simulink model "Main_Sim"  (R2020b)
settings: Solver=FixedStepAuto  StartTime=0.0  StopTime=57060  FixedStep=simParams.sample_time_s  RelTol=1e-3  EnableMultiTasking=on
values from neighbouring files (symbols this model uses):
  test_data = struct    [sim_init.m]
undefined symbols (not defined in the file or in its folder): eclipse, elev_gs_rad, elev_targ_rad, FSW_Lib, gnc_mode, gyro_body_radps, gyro_meas_valid, mag_body_T, mag_meas_valid, mekf_3sigma_rad, mekf_bias_radps, mtq_cmd_Am2, photodiodes_A, rwa_cmd_rpm, sc_above_gs, sc_above_targ, sc_body_rates_radps, sc_quat, Sensors_Lib, sgp4_flag, simParams, solar_panel_power_W, sun_meas_ss_deg, sun_meas_valid, target_gen_flag
libraries: dspstat3 x4, gyroscope_lib x3, magnetometer_lib x3, simulink_extras x2, actuators_lib x1, CDH_command_lib x1, Environment_lib x1, MEKF_Conversion_lib x1, MEKF_lib x1, actuator_processing_lib x1, control_command_generation_lib x1, evironmentEstimation_lib x1
settings Model: Creator=devantormey  LastModifiedBy=Zach Daniel
settings DataIOCC: ReturnWorkspaceOutputs=off
settings OptimizationCC: DefaultParameterBehavior=Inlined  UseDivisionForNetSlopeComputation=on  UseFloatMulNetSlope=on  InlineInvariantSignals=on  PassReuseOutputArgsAs=Individual arguments  ZeroExternalMemoryAtStartup=off  ZeroInternalMemoryAtStartup=off  NoFixptDivByZeroProtection=on  EfficientFloat2IntCast=on  LifeSpan=1  OptimizeBlockOrder=speed  DifferentSizesBufferReuse=on  EfficientTunableParamExpr=on
settings DebuggingCC: ParameterTunabilityLossMsg=error  BusObjectLabelMismatch=error  SFUnexpectedBacktrackingDiag=warning  SFNoUnconditionalDefaultTransitionDiag=warning  ArithmeticOperatorsInVariantConditions=warning
settings HardwareCC: ProdBitPerPointer=32  ProdBitPerSizeT=32  ProdBitPerPtrDiffT=32  ProdLargestAtomicInteger=Long  ProdLargestAtomicFloat=Double  ProdWordSize=32  ProdLongLongMode=on  ProdHWDeviceType=NXP->Cortex-M4
settings SFSimCC: SimUseLocalCustomCode=off  MATLABDynamicMemAlloc=off  CustomCodeUndefinedFunction=UseInterfaceOnly
settings RTWCC: Description=Embedded Coder  SystemTargetFile=ert.tlc  TemplateMakefile=ert_default_tmf  GenerateReport=on  RTWUseLocalCustomCode=off  IncludeHyperlinkInReport=on  LaunchReport=on  GenerateTraceInfo=on  GenerateTraceReport=on  GenerateTraceReportSl=on  GenerateTraceReportSf=on  GenerateTraceReportEml=on  GenerateCodeMetricsReport=on
settings CodeAppCC: ForceParamTrailComments=on  IgnoreCustomStorageClasses=off  OperatorAnnotations=on  SimulinkDataObjDesc=on  SFDataObjDesc=on  CustomSymbolStrGlobalVar=rt$N$M  CustomSymbolStrType=$N$M  CustomSymbolStrFcn=$N$M$F  CustomSymbolStrMacro=$N$M  InsertBlockDesc=on
settings ERTTargetCC: GenerateSampleERTMain=on  IncludeMdlTerminateFcn=off  CombineSignalStateStructs=on  SupportComplex=off  SupportContinuousTime=on  SupportNonInlinedSFcns=on  InlinedParameterPlacement=NonHierarchical  ERTCustomFileTemplate=example_file_process.tlc
settings ConfigComp: CovMetricSettings=dw  CovSaveCumulativeToWorkspaceVar=on  CovSaveSingleToWorkspaceVar=on  CovExternalEMLEnable=off

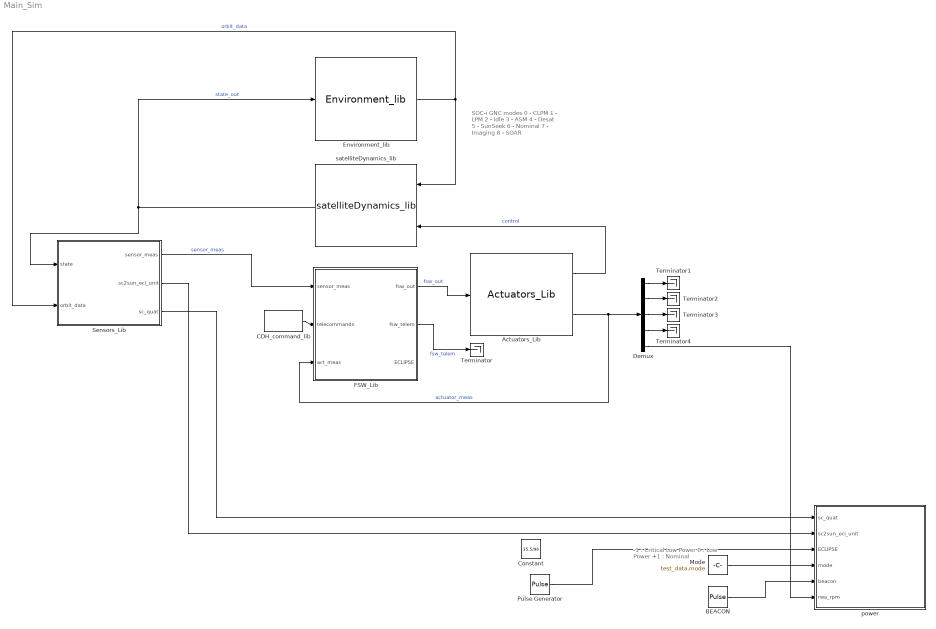
== system Main_Sim ==
  note: SOC-i GNC modes
      | 0 - CLPM
      | 1 - LPM
      | 2 - Idle
      | 3 - ASM
      | 4 - Desat
      | 5 - SunSeek
      | 6 - Nominal
      | 7 - Imaging
      | 8 - SOAR
  note: -1	: Critical Low Power
      |   0	: Low Power
      | +1	: Nominal
  Actuators_Lib : actuators_lib/Actuators_Lib  SystemSampleTime=-1  VariantActivationTime=update diagram  Latency=0  AutoFrameSizeCalculation=off
  BEACON : DiscretePulseGenerator  PulseType=Time based  Period=60  PulseWidth=100 * (1.0 / 60)
  CDH_command_lib : CDH_command_lib/CDH_command_lib  target_lat_deg=target_lat_deg  target_lon_deg=target_lon_deg  target_alt_m=target_alt_m  override_autonomy=0  enable_pointing=off  force_clpm=off  force_lpm=off  enable_img=off  enable_soar=off  triad_override=off  mask{target_lat_deg=44.0, target_lon_deg=-76.5, target_alt_m=0.0, override_autonomy=0, enable_pointing=off, force_clpm=off, force_lpm=off, enable_img=off, enable_soar=off, triad_override=off}
      mask prompts: target_lat_deg "Target Latitude [deg]"; target_lon_deg "Target Longitude [deg]"; target_alt_m "Target Alt [m]"; override_autonomy "Override Autonomous Mode Selection"; enable_pointing "Enable Autonomous Pointing"; force_clpm "CLPM Operating Mode"; force_lpm "LPM Operating Mode"; enable_img "Enable IMG"; enable_soar "Enable SOAR"; triad_override "TRIAD Override"
      mask TypeOptions target_lat_deg: target_lat_deg
      mask TypeOptions target_lon_deg: target_lon_deg
      mask TypeOptions target_alt_m: target_alt_m
      mask TypeOptions override_autonomy: override_autonomy
      mask TypeOptions enable_pointing: enable_pointing
      mask TypeOptions force_clpm: force_clpm
      mask TypeOptions force_lpm: force_lpm
      mask TypeOptions enable_img: enable_img
      mask TypeOptions enable_soar: enable_soar
      mask TypeOptions triad_override: triad_override
      mask DialogControl DescGroupVar Prompt: SOC-i Telecommand Module
      mask DialogControl DescTextVar Prompt: Adjust the parameters that can enter the GNC flight software from the rest of the satellite, including the other subsystems onboard and those that come from the ground station.
  Constant : Constant  Value=35.5/96  VectorParams1D=off
  Demux : Demux  Outputs=[5 4 1 1 4]
  Environment_lib : Environment_lib/Environment_lib  SystemSampleTime=-1  VariantActivationTime=update diagram  Latency=0  AutoFrameSizeCalculation=off
  FSW_Lib : Subsystem  AncestorBlock=FSW_Lib/FSW_Lib
  Mode : Constant  Value=test_data.mode
  Pulse Generator : DiscretePulseGenerator  PulseType=Time based  Period=5760  PulseWidth=100*(35.5/96)
  Sensors_Lib : Subsystem  AncestorBlock=Sensors_Lib/Sensors_Lib
  Terminator{,1..4} (5 alike) : Terminator
  power : Subsystem
  satelliteDynamics_lib : satelliteDynamics_lib/satelliteDynamics_lib  SystemSampleTime=-1  VariantActivationTime=update diagram  Latency=0  AutoFrameSizeCalculation=off
  wires:
  FSW_Lib/1(fsw_out) -> Actuators_Lib/1  "fsw_out"
  Sensors_Lib/1(sensor_meas) -> FSW_Lib/1(sensor_meas)  "sensor_meas"
  satelliteDynamics_lib/1 -> Environment_lib/1, Sensors_Lib/1(state)  "state_out"
  Environment_lib/1 -> Sensors_Lib/2(orbit_data), satelliteDynamics_lib/1  "orbit_data"
  Actuators_Lib/1 -> satelliteDynamics_lib/2  "control"
  CDH_command_lib/1 -> FSW_Lib/2(telecommands)
  Actuators_Lib/2 -> FSW_Lib/3(act_meas), Demux/1  "actuator_meas"
  FSW_Lib/2(fsw_telem) -> Terminator/1  "fsw_telem"
  Mode/1 -> power/4(mode)
  Sensors_Lib/3(sc_quat) -> power/1(sc_quat)
  BEACON/1 -> power/5(beacon)
  Sensors_Lib/2(sc2sun_eci_unit) -> power/2(sc2sun_eci_unit)
  Demux/1 -> Terminator1/1
  Demux/2 -> Terminator2/1
  Demux/3 -> Terminator3/1
  Demux/4 -> Terminator4/1
  Demux/5 -> power/6(rwa_rpm)
  Pulse Generator/1 -> power/3(ECLIPSE)

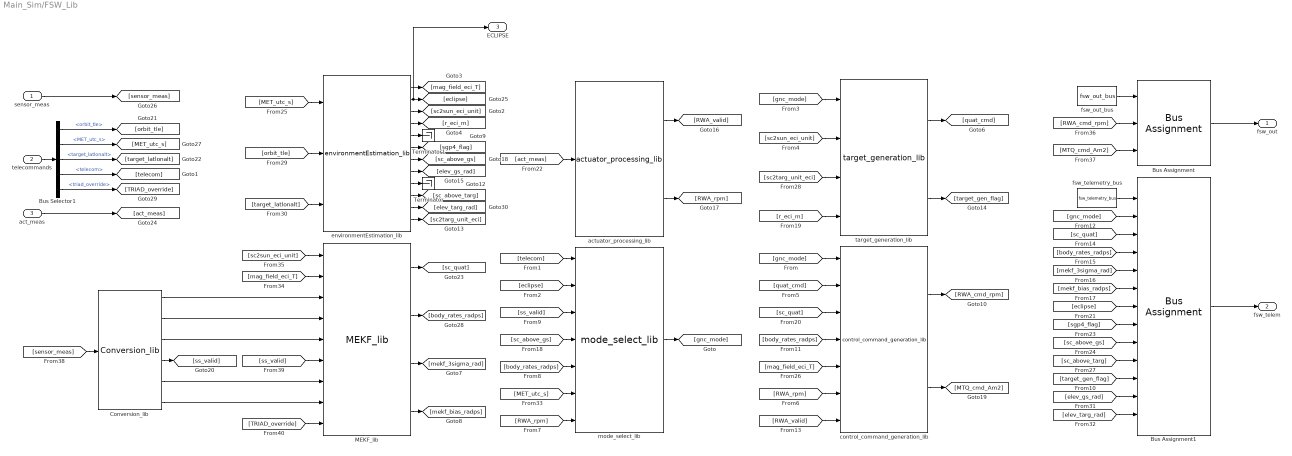
== system Main_Sim/FSW_Lib ==
  sensor_meas : Inport  OutDataTypeStr=Bus: sensor_bus
  telecommands : Inport  Port=2  OutDataTypeStr=Bus: cdh_data
  act_meas : Inport  Port=3  OutDataTypeStr=Bus: actuator_meas
  Bus Assignment : BusAssignment  AssignedSignals=rwa_cmd_rpm,mtq_cmd_Am2
  Bus Assignment1 : BusAssignment  AssignedSignals=gnc_mode,sc_quat,sc_body_rates_radps,mekf_3sigma_rad,mekf_bias_radps,eclipse,sgp4_flag,sc_above_gs,sc_above_targ,target_gen_flag,elev_gs_rad,elev_targ_rad
  Bus Selector1 : BusSelector  OutputSignals=orbit_tle,MET_utc_s,target_latlonalt,telecom,triad_override
  Conversion_lib : MEKF_Conversion_lib/Conversion_lib  SystemSampleTime=-1  VariantActivationTime=update diagram  Latency=0  AutoFrameSizeCalculation=off
  MEKF_lib : MEKF_lib/MEKF_lib  SystemSampleTime=-1  VariantActivationTime=update diagram  Latency=0  AutoFrameSizeCalculation=off
  Terminator : Terminator
  Terminator1 : Terminator
  actuator_processing_lib : actuator_processing_lib/actuator_processing_lib  SystemSampleTime=-1  VariantActivationTime=update diagram  Latency=0  AutoFrameSizeCalculation=off
      link override Rate Transition5: InitialCondition=10
  control_command_generation_lib : control_command_generation_lib/control_command_generation_lib  SystemSampleTime=-1  VariantActivationTime=update diagram  Latency=0  AutoFrameSizeCalculation=off
  environmentEstimation_lib : evironmentEstimation_lib/environmentEstimation_lib  SystemSampleTime=-1  VariantActivationTime=update diagram  Latency=0  AutoFrameSizeCalculation=off
  fsw_out_bus : fsw_out_bus/fsw_out_bus  SystemSampleTime=-1  VariantActivationTime=update diagram  Latency=0  AutoFrameSizeCalculation=off
  fsw_telemetry_bus : fsw_telemetry_bus/fsw_telemetry_bus  SystemSampleTime=-1  VariantActivationTime=update diagram  Latency=0  AutoFrameSizeCalculation=off
  mode_select_lib : mode_select_lib/mode_select_lib  SystemSampleTime=-1  VariantActivationTime=update diagram  Latency=0  AutoFrameSizeCalculation=off
  target_generation_lib : target_gen_lib/target_generation_lib  SystemSampleTime=-1  VariantActivationTime=update diagram  Latency=0  AutoFrameSizeCalculation=off
  fsw_out : Outport  OutDataTypeStr=Bus: fsw_out  VectorParamsAs1DForOutWhenUnconnected=off
  fsw_telem : Outport  Port=2  OutDataTypeStr=Bus: fsw_telemetry  VectorParamsAs1DForOutWhenUnconnected=off
  ECLIPSE : Outport  Port=3  VectorParamsAs1DForOutWhenUnconnected=off
  wires:
  [elev_targ_rad] -> Bus Assignment1/13
  [elev_gs_rad] -> Bus Assignment1/12
  [target_gen_flag] -> Bus Assignment1/11
  [body_rates_radps] -> Bus Assignment1/4
  [sc_above_targ] -> Bus Assignment1/10
  [sc_above_gs] -> Bus Assignment1/9
  [sgp4_flag] -> Bus Assignment1/8
  [eclipse] -> Bus Assignment1/7
  [mekf_bias_radps] -> Bus Assignment1/6
  [mekf_3sigma_rad] -> Bus Assignment1/5
  [sc_quat] -> Bus Assignment1/3
  [gnc_mode] -> Bus Assignment1/2
  fsw_telemetry_bus/1 -> Bus Assignment1/1
  Bus Assignment1/1 -> fsw_telem/1
  actuator_processing_lib/1 -> [RWA_valid]
  [sc2sun_eci_unit] -> target_generation_lib/2
  [gnc_mode] -> target_generation_lib/1
  [sc2targ_unit_eci] -> target_generation_lib/3
  [r_eci_m] -> target_generation_lib/4
  target_generation_lib/1 -> [quat_cmd]
  target_generation_lib/2 -> [target_gen_flag]
  control_command_generation_lib/2 -> [MTQ_cmd_Am2]
  control_command_generation_lib/1 -> [RWA_cmd_rpm]
  [quat_cmd] -> control_command_generation_lib/2
  [gnc_mode] -> control_command_generation_lib/1
  [sc_quat] -> control_command_generation_lib/3
  [body_rates_radps] -> control_command_generation_lib/4
  [RWA_rpm] -> control_command_generation_lib/6
  [RWA_valid] -> control_command_generation_lib/7
  [mag_field_eci_T] -> control_command_generation_lib/5
  environmentEstimation_lib/10 -> [sc_above_targ]
  environmentEstimation_lib/8 -> [elev_gs_rad]
  environmentEstimation_lib/7 -> [sc_above_gs]
  environmentEstimation_lib/6 -> [sgp4_flag]
  environmentEstimation_lib/5 -> Terminator1/1
  environmentEstimation_lib/4 -> [r_eci_m]
  [ss_valid] -> MEKF_lib/6
  [MTQ_cmd_Am2] -> Bus Assignment/3
  [RWA_cmd_rpm] -> Bus Assignment/2
  fsw_out_bus/1 -> Bus Assignment/1
  [sensor_meas] -> Conversion_lib/1
  sensor_meas/1 -> [sensor_meas]
  MEKF_lib/4 -> [mekf_bias_radps]
  MEKF_lib/3 -> [mekf_3sigma_rad]
  MEKF_lib/2 -> [body_rates_radps]
  MEKF_lib/1 -> [sc_quat]
  [TRIAD_override] -> MEKF_lib/9
  [mag_field_eci_T] -> MEKF_lib/2
  [sc2sun_eci_unit] -> MEKF_lib/1
  Conversion_lib/1 -> MEKF_lib/3
  Conversion_lib/2 -> MEKF_lib/4
  Conversion_lib/3 -> MEKF_lib/5
  Conversion_lib/4 -> [ss_valid]
  Conversion_lib/5 -> MEKF_lib/7
  Conversion_lib/6 -> MEKF_lib/8
  telecommands/1 -> Bus Selector1/1
  Bus Assignment/1 -> fsw_out/1
  mode_select_lib/1 -> [gnc_mode]
  [telecom] -> mode_select_lib/1
  [eclipse] -> mode_select_lib/2
  [sc_above_gs] -> mode_select_lib/4
  [body_rates_radps] -> mode_select_lib/5
  [RWA_rpm] -> mode_select_lib/7
  [ss_valid] -> mode_select_lib/3
  environmentEstimation_lib/1 -> [mag_field_eci_T]
  environmentEstimation_lib/2 -> ECLIPSE/1, [eclipse]
  environmentEstimation_lib/3 -> [sc2sun_eci_unit]
  environmentEstimation_lib/9 -> Terminator/1
  [MET_utc_s] -> environmentEstimation_lib/1
  [orbit_tle] -> environmentEstimation_lib/2
  act_meas/1 -> [act_meas]
  actuator_processing_lib/2 -> [RWA_rpm]
  [act_meas] -> actuator_processing_lib/1
  environmentEstimation_lib/12 -> [sc2targ_unit_eci]
  environmentEstimation_lib/11 -> [elev_targ_rad]
  Bus Selector1/2 -> [MET_utc_s]  "<MET_utc_s>"
  Bus Selector1/1 -> [orbit_tle]  "<orbit_tle>"
  Bus Selector1/3 -> [target_latlonalt]  "<target_latlonalt>"
  [target_latlonalt] -> environmentEstimation_lib/3
  [MET_utc_s] -> mode_select_lib/6
  Bus Selector1/4 -> [telecom]  "<telecom>"
  Bus Selector1/5 -> [TRIAD_override]  "<triad_override>"

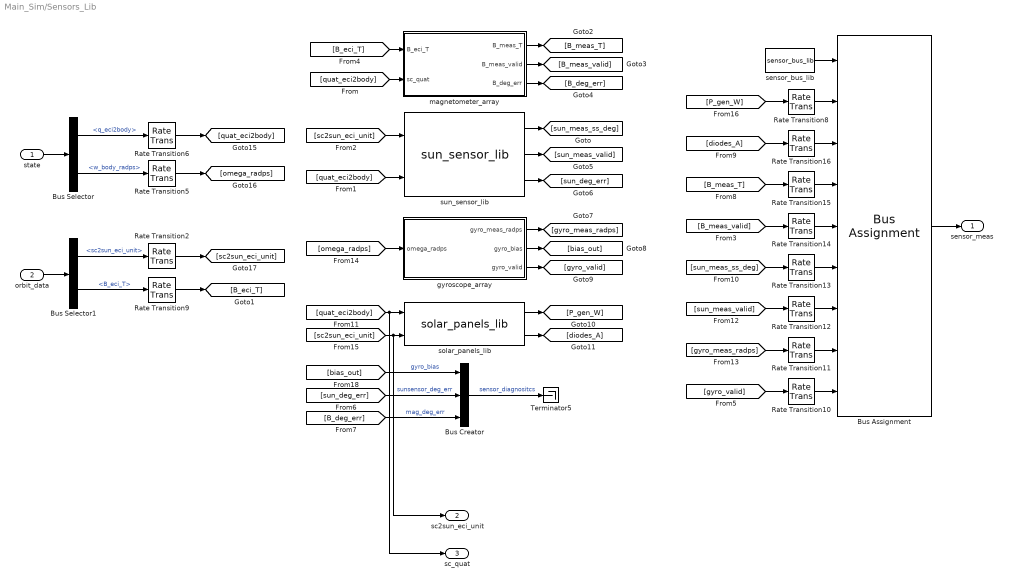
== system Main_Sim/Sensors_Lib ==
  state : Inport  OutDataTypeStr=Bus: state
  orbit_data : Inport  Port=2  OutDataTypeStr=Bus: orbit_data
  Bus Assignment : BusAssignment  AssignedSignals=solar_panel_power_W,photodiodes_A,mag_body_T,mag_meas_valid,sun_meas_ss_deg,sun_meas_valid,gyro_body_radps,gyro_meas_valid
  Bus Creator : BusCreator  Inputs=3
  Bus Selector : BusSelector  OutputSignals=q_eci2body,w_body_radps
  Bus Selector1 : BusSelector  OutputSignals=sc2sun_eci_unit,B_eci_T
  Rate Transition{2,6,8..16} (11 alike) : RateTransition  OutPortSampleTime=simParams.sensors.sample_time_s
  Rate Transition5 : RateTransition  InitialCondition=50  OutPortSampleTime=simParams.sensors.sample_time_s
  Terminator5 : Terminator
  gyroscope_array : Subsystem
  magnetometer_array : Subsystem
  sensor_bus_lib : sensor_bus/sensor_bus_lib  SystemSampleTime=-1  VariantActivationTime=update diagram  Latency=0  AutoFrameSizeCalculation=off
  solar_panels_lib : solar_panels_lib/solar_panels_lib  SystemSampleTime=-1  VariantActivationTime=update diagram  Latency=0  AutoFrameSizeCalculation=off
  "sun_sensor_lib " : sun_sensor_lib/sun_sensor_lib   SystemSampleTime=-1  VariantActivationTime=update diagram  Latency=0  AutoFrameSizeCalculation=off
  sensor_meas : Outport  OutDataTypeStr=Bus: sensor_bus  VectorParamsAs1DForOutWhenUnconnected=off
  sc2sun_eci_unit : Outport  Port=2  VectorParamsAs1DForOutWhenUnconnected=off
  sc_quat : Outport  Port=3  VectorParamsAs1DForOutWhenUnconnected=off
  wires:
  state/1 -> Bus Selector/1
  [diodes_A] -> Rate Transition16/1
  Rate Transition16/1 -> Bus Assignment/3
  Rate Transition8/1 -> Bus Assignment/2
  Rate Transition15/1 -> Bus Assignment/4
  Rate Transition14/1 -> Bus Assignment/5
  Rate Transition13/1 -> Bus Assignment/6
  Rate Transition12/1 -> Bus Assignment/7
  Rate Transition11/1 -> Bus Assignment/8
  Rate Transition10/1 -> Bus Assignment/9
  solar_panels_lib/2 -> [diodes_A]
  Bus Creator/1 -> Terminator5/1  "sensor_diagnositcs"
  [B_deg_err] -> Bus Creator/3  "mag_deg_err"
  [sun_deg_err] -> Bus Creator/2  "sunsensor_deg_err"
  [bias_out] -> Bus Creator/1  "gyro_bias"
  [gyro_valid] -> Rate Transition10/1
  [gyro_meas_radps] -> Rate Transition11/1
  [sun_meas_valid] -> Rate Transition12/1
  [sun_meas_ss_deg] -> Rate Transition13/1
  [B_meas_valid] -> Rate Transition14/1
  [P_gen_W] -> Rate Transition8/1
  [B_meas_T] -> Rate Transition15/1
  solar_panels_lib/1 -> [P_gen_W]
  [quat_eci2body] -> sc_quat/1, solar_panels_lib/1
  [sc2sun_eci_unit] -> sc2sun_eci_unit/1, solar_panels_lib/2
  Rate Transition2/1 -> [sc2sun_eci_unit]
  Bus Selector1/1 -> Rate Transition2/1  "<sc2sun_eci_unit>"
  Rate Transition9/1 -> [B_eci_T]
  Bus Selector1/2 -> Rate Transition9/1  "<B_eci_T>"
  Rate Transition6/1 -> [quat_eci2body]
  Bus Selector/1 -> Rate Transition6/1  "<q_eci2body>"
  Rate Transition5/1 -> [omega_radps]
  gyroscope_array/3(gyro_valid) -> [gyro_valid]
  gyroscope_array/2(gyro_bias) -> [bias_out]
  gyroscope_array/1(gyro_meas_radps) -> [gyro_meas_radps]
  "sun_sensor_lib "/3 -> [sun_deg_err]
  "sun_sensor_lib "/2 -> [sun_meas_valid]
  "sun_sensor_lib "/1 -> [sun_meas_ss_deg]
  magnetometer_array/3(B_deg_err) -> [B_deg_err]
  magnetometer_array/2(B_meas_valid) -> [B_meas_valid]
  magnetometer_array/1(B_meas_T) -> [B_meas_T]
  sensor_bus_lib/1 -> Bus Assignment/1
  [B_eci_T] -> magnetometer_array/1(B_eci_T)
  [sc2sun_eci_unit] -> "sun_sensor_lib "/1
  orbit_data/1 -> Bus Selector1/1
  [omega_radps] -> gyroscope_array/1(omega_radps)
  [quat_eci2body] -> "sun_sensor_lib "/2
  [quat_eci2body] -> magnetometer_array/2(sc_quat)
  Bus Assignment/1 -> sensor_meas/1
  Bus Selector/2 -> Rate Transition5/1  "<w_body_radps>"

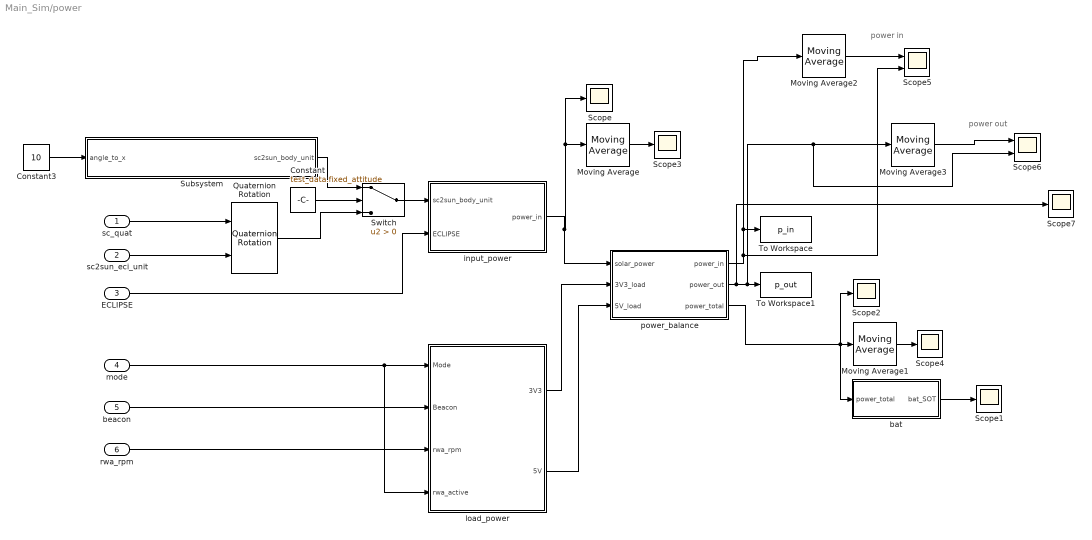
== system Main_Sim/power ==
  note: power out
  note: power in
  sc_quat : Inport
  sc2sun_eci_unit : Inport  Port=2
  ECLIPSE : Inport  Port=3
  mode : Inport  Port=4
  beacon : Inport  Port=5
  rwa_rpm : Inport  Port=6
  Constant : Constant  Value=test_data.fixed_attitude
  Constant3 : Constant  Value=10
  Moving Average : dspstat3/Moving Average  Method=Exponential weighting  ForgettingFactorPort=off  SpecifyWindowLength=on  WindowLength=4  ForgettingFactor=1.0  SimulateUsing=Code generation
  Moving Average1 : dspstat3/Moving Average  Method=Exponential weighting  ForgettingFactorPort=off  SpecifyWindowLength=on  WindowLength=4  ForgettingFactor=1.0  SimulateUsing=Code generation
  Moving Average2 : dspstat3/Moving Average  Method=Exponential weighting  ForgettingFactorPort=off  SpecifyWindowLength=on  WindowLength=4  ForgettingFactor=1  SimulateUsing=Code generation
  Moving Average3 : dspstat3/Moving Average  Method=Exponential weighting  ForgettingFactorPort=off  SpecifyWindowLength=on  WindowLength=4  ForgettingFactor=1  SimulateUsing=Code generation
  Quaternion Rotation : aerolibutil/Quaternion Rotation
  Scope{,1..4,7} (6 alike) : Scope
  Scope5 : Scope  NumInputPorts=2
  Scope6 : Scope  NumInputPorts=2
  Subsystem : Subsystem
  Switch : Switch  Criteria=u2 > Threshold
  To Workspace : ToWorkspace  VariableName=p_in  SampleTime=-1
  To Workspace1 : ToWorkspace  VariableName=p_out  SampleTime=-1
  bat : Subsystem
  input_power : Subsystem
  load_power : Subsystem
  power_balance : Subsystem
  wires:
  load_power/1(3V3) -> power_balance/2("3V3_load ")
  input_power/1(power_in) -> power_balance/1(solar_power), Moving Average/1, Scope/1
  rwa_rpm/1 -> load_power/3(rwa_rpm)
  mode/1 -> load_power/4(rwa_active), load_power/1(Mode)
  beacon/1 -> load_power/2(Beacon)
  Moving Average1/1 -> Scope4/1
  load_power/2(5V) -> power_balance/3(5V_load)
  bat/1(bat_SOT) -> Scope1/1
  Moving Average/1 -> Scope3/1
  sc_quat/1 -> Quaternion Rotation/1
  sc2sun_eci_unit/1 -> Quaternion Rotation/2
  ECLIPSE/1 -> input_power/2(ECLIPSE)
  power_balance/3(power_total) -> Scope2/1, bat/1(power_total), Moving Average1/1
  power_balance/1(power_in) -> Scope5/2, Moving Average2/1, To Workspace/1
  Constant3/1 -> Subsystem/1(angle_to_x)
  Constant/1 -> Switch/2
  Subsystem/1(sc2sun_body_unit) -> Switch/1
  Quaternion Rotation/1 -> Switch/3
  Switch/1 -> input_power/1(sc2sun_body_unit)
  power_balance/2(power_out) -> Scope7/1, Scope6/2, Moving Average3/1, To Workspace1/1
  Moving Average2/1 -> Scope5/1
  Moving Average3/1 -> Scope6/1

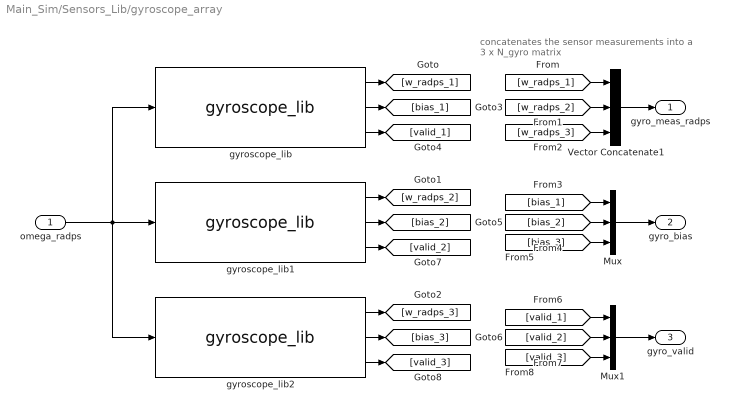
== system Main_Sim/Sensors_Lib/gyroscope_array ==
  note: concatenates the sensor measurements
      | into a 3 x N_gyro matrix
  omega_radps : Inport
  Mux : Mux  Inputs=3
  Mux1 : Mux  Inputs=3
  Vector Concatenate1 : Concatenate  NumInputs=3  Mode=Multidimensional array  ConcatenateDimension=2
  gyroscope_lib : gyroscope_lib/gyroscope_lib  id_s=1
  gyroscope_lib1 : gyroscope_lib/gyroscope_lib  id_s=2
  gyroscope_lib2 : gyroscope_lib/gyroscope_lib  id_s=3
  gyro_meas_radps : Outport  VectorParamsAs1DForOutWhenUnconnected=off
  gyro_bias : Outport  Port=2  VectorParamsAs1DForOutWhenUnconnected=off
  gyro_valid : Outport  Port=3  VectorParamsAs1DForOutWhenUnconnected=off
  wires:
  [valid_3] -> Mux1/3
  [valid_2] -> Mux1/2
  [valid_1] -> Mux1/1
  Mux1/1 -> gyro_valid/1
  [bias_3] -> Mux/3
  [bias_2] -> Mux/2
  [bias_1] -> Mux/1
  Mux/1 -> gyro_bias/1
  [w_radps_3] -> Vector Concatenate1/3
  [w_radps_2] -> Vector Concatenate1/2
  [w_radps_1] -> Vector Concatenate1/1
  Vector Concatenate1/1 -> gyro_meas_radps/1
  gyroscope_lib2/3 -> [valid_3]
  gyroscope_lib1/3 -> [valid_2]
  gyroscope_lib2/2 -> [bias_3]
  gyroscope_lib1/2 -> [bias_2]
  gyroscope_lib/3 -> [valid_1]
  gyroscope_lib/2 -> [bias_1]
  gyroscope_lib2/1 -> [w_radps_3]
  gyroscope_lib1/1 -> [w_radps_2]
  gyroscope_lib/1 -> [w_radps_1]
  omega_radps/1 -> gyroscope_lib1/1, gyroscope_lib/1, gyroscope_lib2/1

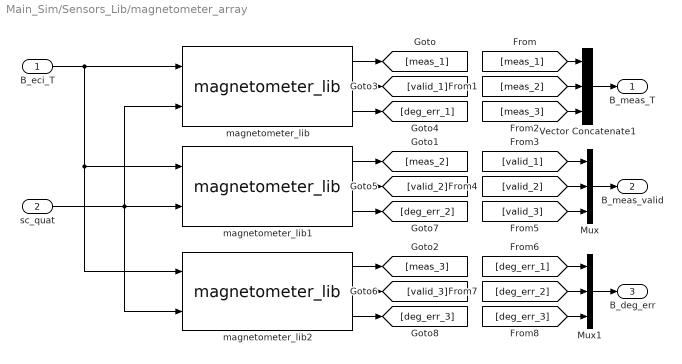
== system Main_Sim/Sensors_Lib/magnetometer_array ==
  B_eci_T : Inport
  sc_quat : Inport  Port=2
  Mux : Mux  Inputs=3
  Mux1 : Mux  Inputs=3
  Vector Concatenate1 : Concatenate  NumInputs=3  Mode=Multidimensional array  ConcatenateDimension=2
  magnetometer_lib : magnetometer_lib/magnetometer_lib  id_s=1
  magnetometer_lib1 : magnetometer_lib/magnetometer_lib  id_s=2
  magnetometer_lib2 : magnetometer_lib/magnetometer_lib  id_s=1
  B_meas_T : Outport  VectorParamsAs1DForOutWhenUnconnected=off
  B_meas_valid : Outport  Port=2  VectorParamsAs1DForOutWhenUnconnected=off
  B_deg_err : Outport  Port=3  VectorParamsAs1DForOutWhenUnconnected=off
  wires:
  [deg_err_3] -> Mux1/3
  [deg_err_2] -> Mux1/2
  [deg_err_1] -> Mux1/1
  Mux1/1 -> B_deg_err/1
  [valid_3] -> Mux/3
  [valid_2] -> Mux/2
  [valid_1] -> Mux/1
  Mux/1 -> B_meas_valid/1
  [meas_3] -> Vector Concatenate1/3
  [meas_2] -> Vector Concatenate1/2
  [meas_1] -> Vector Concatenate1/1
  Vector Concatenate1/1 -> B_meas_T/1
  magnetometer_lib2/3 -> [deg_err_3]
  magnetometer_lib1/3 -> [deg_err_2]
  magnetometer_lib2/2 -> [valid_3]
  magnetometer_lib1/2 -> [valid_2]
  magnetometer_lib/3 -> [deg_err_1]
  magnetometer_lib/2 -> [valid_1]
  magnetometer_lib2/1 -> [meas_3]
  magnetometer_lib1/1 -> [meas_2]
  magnetometer_lib/1 -> [meas_1]
  B_eci_T/1 -> magnetometer_lib1/1, magnetometer_lib2/1, magnetometer_lib/1
  sc_quat/1 -> magnetometer_lib1/2, magnetometer_lib2/2, magnetometer_lib/2

== system Main_Sim/power/Subsystem ==
  angle_to_x : Inport
  Constant1 : Constant  Value=90
  Constant2 : Constant  Value=0
  Cos : Trigonometry  Operator=cos
  Cos1 : Trigonometry  Operator=cos
  Degrees to Radians : simulink_extras/Transformations/Degrees to Radians
  Degrees to Radians1 : simulink_extras/Transformations/Degrees to Radians
  Mux : Mux  Inputs=3
  Subtract : Sum  Inputs=+-
  sc2sun_body_unit : Outport  VectorParamsAs1DForOutWhenUnconnected=off
  wires:
  Subtract/1 -> Degrees to Radians1/1
  Constant2/1 -> Mux/3
  Cos1/1 -> Mux/2
  Degrees to Radians1/1 -> Cos1/1
  Degrees to Radians/1 -> Cos/1
  Cos/1 -> Mux/1
  Mux/1 -> sc2sun_body_unit/1
  Constant1/1 -> Subtract/1
  angle_to_x/1 -> Subtract/2, Degrees to Radians/1

== system Main_Sim/power/bat ==
  power_total : Inport
  Constant4 : Constant  Value=1/(60*60)
  Constant5 : Constant  Value=20000
  Divide : Product  Inputs=*/
  Integrator : Integrator  InitialCondition=20000  LimitOutput=on  UpperSaturationLimit=20000  LowerSaturationLimit=0
  Product : Product
  bat_SOT : Outport  VectorParamsAs1DForOutWhenUnconnected=off
  wires:
  Constant4/1 -> Product/2
  Constant5/1 -> Divide/2
  power_total/1 -> Product/1
  Product/1 -> Integrator/1
  Integrator/1 -> Divide/1
  Divide/1 -> bat_SOT/1

== system Main_Sim/power/input_power ==
  sc2sun_body_unit : Inport
  ECLIPSE : Inport  Port=2
  Constant1 : Constant
  Product : Product
  Subtract : Sum  Inputs=+-
  Sum of Elements : Sum  Inputs=+
  Terminator : Terminator
  solar_panel_power : MATLAB Function  TreatAsAtomicUnit=on
  power_in : Outport  VectorParamsAs1DForOutWhenUnconnected=off
  wires:
  Product/1 -> Sum of Elements/1
  solar_panel_power/2(diodes_A) -> Terminator/1
  solar_panel_power/1(power_gen_W) -> Product/1
  Sum of Elements/1 -> power_in/1
  sc2sun_body_unit/1 -> solar_panel_power/1(sc2sun_body_unit)
  Constant1/1 -> Subtract/1
  ECLIPSE/1 -> Subtract/2
  Subtract/1 -> Product/2

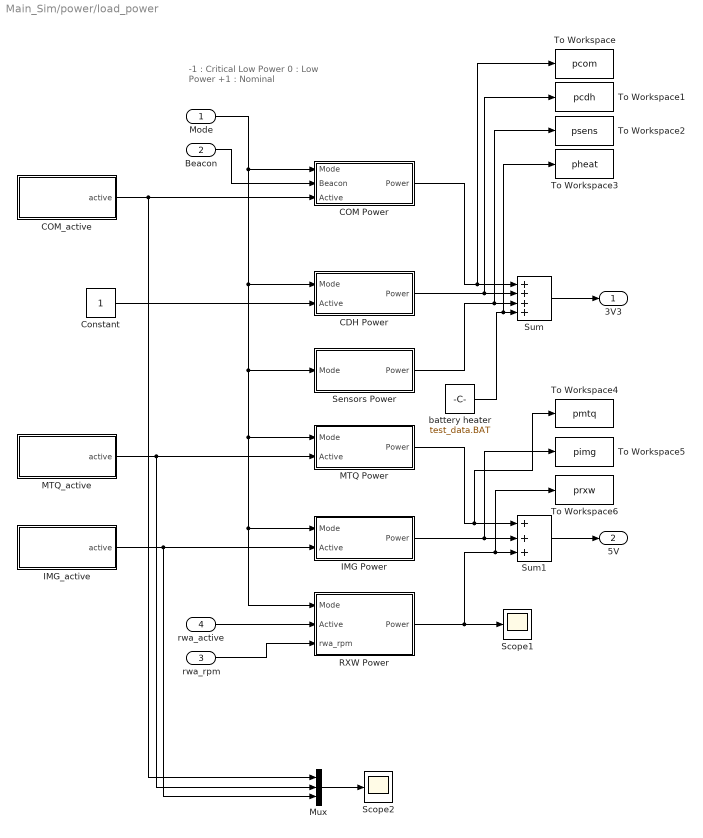
== system Main_Sim/power/load_power ==
  note: -1	: Critical Low Power
      |   0	: Low Power
      | +1	: Nominal
  Mode : Inport
  Beacon : Inport  Port=2
  rwa_rpm : Inport  Port=3
  rwa_active : Inport  Port=4
  CDH Power : Subsystem
  COM Power : Subsystem
  COM_active : Subsystem
  Constant : Constant
  IMG Power : Subsystem
  IMG_active : Subsystem
  MTQ Power : Subsystem
  MTQ_active : Subsystem
  Mux : Mux  Inputs=3
  RXW Power : Subsystem
  Scope1 : Scope
  Scope2 : Scope
  Sensors Power : Subsystem
  Sum : Sum  Inputs=++++
  Sum1 : Sum  Inputs=+++
  To Workspace : ToWorkspace  VariableName=pcom  SampleTime=-1
  To Workspace1 : ToWorkspace  VariableName=pcdh  SampleTime=-1
  To Workspace2 : ToWorkspace  VariableName=psens  SampleTime=-1
  To Workspace3 : ToWorkspace  VariableName=pheat  SampleTime=-1
  To Workspace4 : ToWorkspace  VariableName=pmtq  SampleTime=-1
  To Workspace5 : ToWorkspace  VariableName=pimg  SampleTime=-1
  To Workspace6 : ToWorkspace  VariableName=prxw  SampleTime=-1
  battery heater : Constant  Value=test_data.BAT
  3V3 : Outport  VectorParamsAs1DForOutWhenUnconnected=off
  5V : Outport  Port=2  VectorParamsAs1DForOutWhenUnconnected=off
  wires:
  Mode/1 -> RXW Power/1(Mode), IMG Power/1(Mode), MTQ Power/1(Mode), Sensors Power/1(Mode), CDH Power/1(Mode), COM Power/1(Mode)
  Beacon/1 -> COM Power/2(Beacon)
  rwa_active/1 -> RXW Power/2(Active)
  CDH Power/1(Power) -> Sum/2, To Workspace1/1
  COM Power/1(Power) -> Sum/1, To Workspace/1
  Sensors Power/1(Power) -> Sum/3, To Workspace2/1
  IMG Power/1(Power) -> To Workspace5/1, Sum1/2
  RXW Power/1(Power) -> Scope1/1, To Workspace6/1, Sum1/3
  Sum/1 -> 3V3/1
  Sum1/1 -> 5V/1
  battery heater/1 -> To Workspace3/1, Sum/4
  rwa_rpm/1 -> RXW Power/3(rwa_rpm)
  MTQ Power/1(Power) -> To Workspace4/1, Sum1/1
  IMG_active/1(active) -> Mux/3, IMG Power/2(Active)
  MTQ_active/1(active) -> Mux/2, MTQ Power/2(Active)
  Constant/1 -> CDH Power/2(Active)
  COM_active/1(active) -> Mux/1, COM Power/3("Active ")
  Mux/1 -> Scope2/1

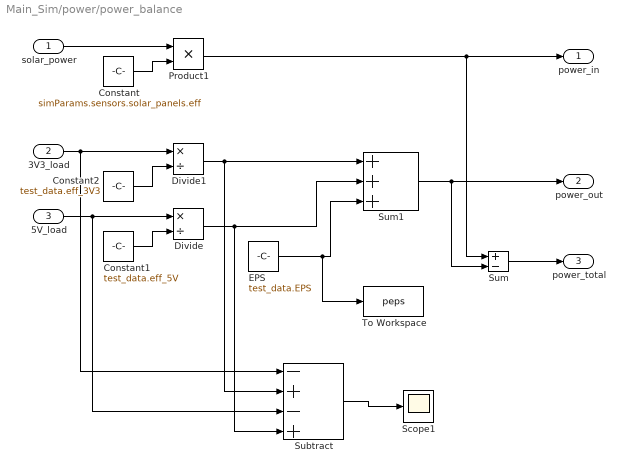
== system Main_Sim/power/power_balance ==
  solar_power : Inport
  "3V3_load " : Inport  Port=2
  5V_load : Inport  Port=3
  Constant : Constant  Value=simParams.sensors.solar_panels.eff
  Constant1 : Constant  Value=test_data.eff_5V
  Constant2 : Constant  Value=test_data.eff_3V3
  Divide : Product  Inputs=*/
  Divide1 : Product  Inputs=*/
  EPS : Constant  Value=test_data.EPS
  Product1 : Product
  Scope1 : Scope
  Subtract : Sum  Inputs=-+-+
  Sum : Sum  Inputs=+-
  Sum1 : Sum  Inputs=+++
  To Workspace : ToWorkspace  VariableName=peps  SampleTime=-1
  power_in : Outport  VectorParamsAs1DForOutWhenUnconnected=off
  power_out : Outport  Port=2  VectorParamsAs1DForOutWhenUnconnected=off
  power_total : Outport  Port=3  VectorParamsAs1DForOutWhenUnconnected=off
  wires:
  solar_power/1 -> Product1/1
  Constant/1 -> Product1/2
  5V_load/1 -> Subtract/3, Divide/1
  Constant1/1 -> Divide/2
  Constant2/1 -> Divide1/2
  "3V3_load "/1 -> Subtract/1, Divide1/1
  Divide1/1 -> Sum1/1, Subtract/2
  Product1/1 -> Sum/1, power_in/1
  Divide/1 -> Sum1/2, Subtract/4
  Sum1/1 -> Sum/2, power_out/1
  EPS/1 -> To Workspace/1, Sum1/3
  Subtract/1 -> Scope1/1
  Sum/1 -> power_total/1

== system Main_Sim/power/load_power/CDH Power ==
  Mode : Inport
  Active : Inport  Port=2
  Constant : Constant  Value=-1
  Constant1 : Constant  Value=test_data.CDH_Idle
  Constant2 : Constant  Value=test_data.CDH_Active
  GreaterThan : RelationalOperator  OutDataTypeStr=boolean  RndMeth=Simplest
  Logical Operator : Logic  AllPortsSameDT=off  OutDataTypeStr=boolean
  Switch : Switch  Criteria=u2 > Threshold
  Power : Outport
  wires:
  Constant/1 -> GreaterThan/2
  Mode/1 -> GreaterThan/1
  GreaterThan/1 -> Logical Operator/1
  Active/1 -> Logical Operator/2
  Logical Operator/1 -> Switch/2
  Switch/1 -> Power/1
  Constant2/1 -> Switch/1
  Constant1/1 -> Switch/3

== system Main_Sim/power/load_power/COM Power ==
  Mode : Inport
  Beacon : Inport  Port=2
  "Active " : Inport  Port=3
  Constant : Constant  Value=0
  Constant1 : Constant  Value=test_data.COM_RX
  Constant2 : Constant  Value=test_data.COM_TX+test_data.COM_RX
  GreaterThan : RelationalOperator  OutDataTypeStr=boolean  RndMeth=Simplest
  Logical Operator : Logic  AllPortsSameDT=off  OutDataTypeStr=boolean
  OR : Logic  Operator=OR  IconShape=distinctive  AllPortsSameDT=off  OutDataTypeStr=boolean
  Switch : Switch  Criteria=u2 > Threshold
  Power : Outport
  wires:
  Constant/1 -> GreaterThan/2
  Mode/1 -> GreaterThan/1
  GreaterThan/1 -> Logical Operator/1
  Constant2/1 -> Switch/1
  Constant1/1 -> Switch/3
  Logical Operator/1 -> Switch/2
  Switch/1 -> Power/1
  Beacon/1 -> OR/1
  "Active "/1 -> OR/2
  OR/1 -> Logical Operator/2

== system Main_Sim/power/load_power/COM_active ==
  Constant : Constant  Value=0
  Constant1 : Constant  Value=test_data.com_en
  Pulse Generator : DiscretePulseGenerator  PulseType=Time based  Period=10  PulseWidth=5
  Switch : Switch  Criteria=u2 > Threshold
  active : Outport  VectorParamsAs1DForOutWhenUnconnected=off
  wires:
  Constant/1 -> Switch/3
  Constant1/1 -> Switch/2
  Switch/1 -> active/1
  Pulse Generator/1 -> Switch/1

== system Main_Sim/power/load_power/IMG Power ==
  Mode : Inport
  Active : Inport  Port=2
  Constant : Constant
  Constant1 : Constant  Value=test_data.IMG_Idle
  Constant2 : Constant  Value=test_data.IMG_Active
  GreaterThan : RelationalOperator  OutDataTypeStr=boolean  RndMeth=Simplest
  Logical Operator : Logic  AllPortsSameDT=off  OutDataTypeStr=boolean
  Switch : Switch  Criteria=u2 > Threshold
  Power : Outport
  wires:
  Constant/1 -> GreaterThan/2
  Mode/1 -> GreaterThan/1
  GreaterThan/1 -> Logical Operator/1
  Active/1 -> Logical Operator/2
  Logical Operator/1 -> Switch/2
  Constant2/1 -> Switch/1
  Constant1/1 -> Switch/3
  Switch/1 -> Power/1

== system Main_Sim/power/load_power/IMG_active ==
  Constant : Constant  Value=0
  Constant1 : Constant  Value=test_data.img_en
  Pulse Generator : DiscretePulseGenerator  PulseType=Time based  Period=5720  PulseWidth=100*(300/5720)  PhaseDelay=400
  Switch : Switch  Criteria=u2 > Threshold
  active : Outport  VectorParamsAs1DForOutWhenUnconnected=off
  wires:
  Constant/1 -> Switch/3
  Constant1/1 -> Switch/2
  Switch/1 -> active/1
  Pulse Generator/1 -> Switch/1

== system Main_Sim/power/load_power/MTQ Power ==
  Mode : Inport
  Active : Inport  Port=2
  Constant : Constant
  Constant1 : Constant  Value=test_data.MTQ_Active
  Constant2 : Constant  Value=test_data.MTQ_Idle
  GreaterThan : RelationalOperator  OutDataTypeStr=boolean  RndMeth=Simplest
  Logical Operator : Logic  AllPortsSameDT=off  OutDataTypeStr=boolean
  Switch : Switch  Criteria=u2 > Threshold
  Power : Outport
  wires:
  Constant/1 -> GreaterThan/2
  Mode/1 -> GreaterThan/1
  GreaterThan/1 -> Logical Operator/1
  Constant1/1 -> Switch/1
  Active/1 -> Logical Operator/2
  Logical Operator/1 -> Switch/2
  Constant2/1 -> Switch/3
  Switch/1 -> Power/1

== system Main_Sim/power/load_power/MTQ_active ==
  Constant : Constant  Value=0
  Constant1 : Constant  Value=test_data.mtq_en
  Pulse Generator : DiscretePulseGenerator  PulseType=Time based  Period=5720  PulseWidth=100*(1200/5720)
  Switch : Switch  Criteria=u2 > Threshold
  active : Outport  VectorParamsAs1DForOutWhenUnconnected=off
  wires:
  Constant/1 -> Switch/3
  Constant1/1 -> Switch/2
  Switch/1 -> active/1
  Pulse Generator/1 -> Switch/1

== system Main_Sim/power/load_power/RXW Power ==
  Mode : Inport
  Active : Inport  Port=2
  rwa_rpm : Inport  Port=3
  Subsystem1 : Subsystem
  Power : Outport
  wires:
  Mode/1 -> Subsystem1/1(Mode)
  Active/1 -> Subsystem1/2(Active)
  rwa_rpm/1 -> Subsystem1/3(RPM)
  Subsystem1/1(Power) -> Power/1

== system Main_Sim/power/load_power/Sensors Power ==
  Mode : Inport
  Constant : Constant  Value=0
  Constant1 : Constant  Value=test_data.SEN_AVG
  GreaterThan : RelationalOperator  OutDataTypeStr=boolean  RndMeth=Simplest
  Product1 : Product
  Power : Outport
  wires:
  Constant/1 -> GreaterThan/2
  Mode/1 -> GreaterThan/1
  GreaterThan/1 -> Product1/2
  Constant1/1 -> Product1/1
  Product1/1 -> Power/1

== system Main_Sim/power/load_power/RXW Power/Subsystem1 ==
  Mode : Inport
  Active : Inport  Port=2
  RPM : Inport  Port=3
  Demux : Demux
  Subsystem : Subsystem
  Subsystem1 : Subsystem
  Subsystem2 : Subsystem
  Subsystem3 : Subsystem
  Sum : Sum  Inputs=++++
  Power : Outport  VectorParamsAs1DForOutWhenUnconnected=off
  wires:
  RPM/1 -> Demux/1
  Mode/1 -> Subsystem3/1(Mode), Subsystem2/1(Mode), Subsystem1/1(Mode), Subsystem/1(Mode)
  Active/1 -> Subsystem3/2(Active), Subsystem2/2(Active), Subsystem1/2(Active), Subsystem/2(Active)
  Demux/1 -> Subsystem/3(RPM)
  Demux/2 -> Subsystem1/3(RPM)
  Demux/3 -> Subsystem2/3(RPM)
  Demux/4 -> Subsystem3/3(RPM)
  Subsystem1/1(Power) -> Sum/2
  Subsystem2/1(Power) -> Sum/3
  Subsystem3/1(Power) -> Sum/4
  Subsystem/1(Power) -> Sum/1
  Sum/1 -> Power/1

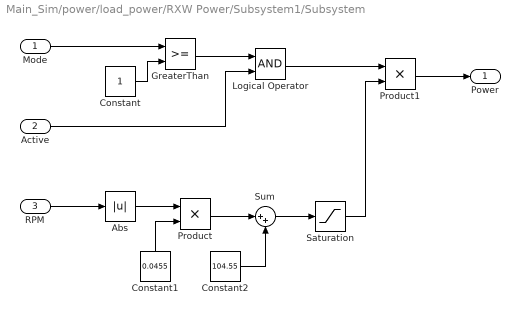
== system Main_Sim/power/load_power/RXW Power/Subsystem1/Subsystem ==
  Mode : Inport
  Active : Inport  Port=2
  RPM : Inport  Port=3
  Abs : Abs
  Constant : Constant
  Constant1 : Constant  Value=0.0455
  Constant2 : Constant  Value=104.55
  GreaterThan : RelationalOperator  OutDataTypeStr=boolean  RndMeth=Simplest
  Logical Operator : Logic  AllPortsSameDT=off  OutDataTypeStr=boolean
  Product : Product
  Product1 : Product
  Saturation : Saturate  UpperLimit=inf  LowerLimit=150
  Sum : Sum  Inputs=|++
  Power : Outport  VectorParamsAs1DForOutWhenUnconnected=off
  wires:
  Constant1/1 -> Product/2
  Logical Operator/1 -> Product1/1
  GreaterThan/1 -> Logical Operator/1
  Mode/1 -> GreaterThan/1
  Active/1 -> Logical Operator/2
  Constant/1 -> GreaterThan/2
  Product/1 -> Sum/1
  Constant2/1 -> Sum/2
  Sum/1 -> Saturation/1
  RPM/1 -> Abs/1
  Abs/1 -> Product/1
  Saturation/1 -> Product1/2
  Product1/1 -> Power/1

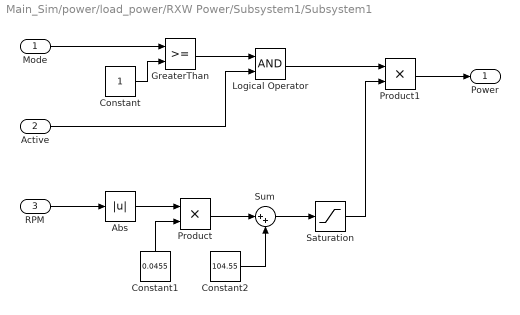
== system Main_Sim/power/load_power/RXW Power/Subsystem1/Subsystem1 ==
  Mode : Inport
  Active : Inport  Port=2
  RPM : Inport  Port=3
  Abs : Abs
  Constant : Constant
  Constant1 : Constant  Value=0.0455
  Constant2 : Constant  Value=104.55
  GreaterThan : RelationalOperator  OutDataTypeStr=boolean  RndMeth=Simplest
  Logical Operator : Logic  AllPortsSameDT=off  OutDataTypeStr=boolean
  Product : Product
  Product1 : Product
  Saturation : Saturate  UpperLimit=inf  LowerLimit=150
  Sum : Sum  Inputs=|++
  Power : Outport  VectorParamsAs1DForOutWhenUnconnected=off
  wires:
  Constant1/1 -> Product/2
  Logical Operator/1 -> Product1/1
  GreaterThan/1 -> Logical Operator/1
  Mode/1 -> GreaterThan/1
  Active/1 -> Logical Operator/2
  Constant/1 -> GreaterThan/2
  Product/1 -> Sum/1
  Constant2/1 -> Sum/2
  Sum/1 -> Saturation/1
  RPM/1 -> Abs/1
  Abs/1 -> Product/1
  Saturation/1 -> Product1/2
  Product1/1 -> Power/1

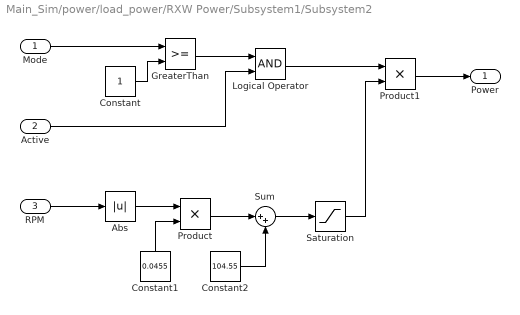
== system Main_Sim/power/load_power/RXW Power/Subsystem1/Subsystem2 ==
  Mode : Inport
  Active : Inport  Port=2
  RPM : Inport  Port=3
  Abs : Abs
  Constant : Constant
  Constant1 : Constant  Value=0.0455
  Constant2 : Constant  Value=104.55
  GreaterThan : RelationalOperator  OutDataTypeStr=boolean  RndMeth=Simplest
  Logical Operator : Logic  AllPortsSameDT=off  OutDataTypeStr=boolean
  Product : Product
  Product1 : Product
  Saturation : Saturate  UpperLimit=inf  LowerLimit=150
  Sum : Sum  Inputs=|++
  Power : Outport  VectorParamsAs1DForOutWhenUnconnected=off
  wires:
  Constant1/1 -> Product/2
  Logical Operator/1 -> Product1/1
  GreaterThan/1 -> Logical Operator/1
  Mode/1 -> GreaterThan/1
  Active/1 -> Logical Operator/2
  Constant/1 -> GreaterThan/2
  Product/1 -> Sum/1
  Constant2/1 -> Sum/2
  Sum/1 -> Saturation/1
  RPM/1 -> Abs/1
  Abs/1 -> Product/1
  Saturation/1 -> Product1/2
  Product1/1 -> Power/1

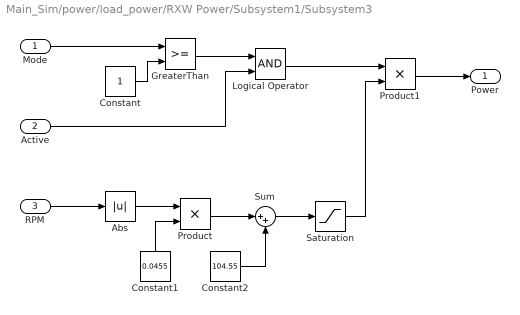
== system Main_Sim/power/load_power/RXW Power/Subsystem1/Subsystem3 ==
  Mode : Inport
  Active : Inport  Port=2
  RPM : Inport  Port=3
  Abs : Abs
  Constant : Constant
  Constant1 : Constant  Value=0.0455
  Constant2 : Constant  Value=104.55
  GreaterThan : RelationalOperator  OutDataTypeStr=boolean  RndMeth=Simplest
  Logical Operator : Logic  AllPortsSameDT=off  OutDataTypeStr=boolean
  Product : Product
  Product1 : Product
  Saturation : Saturate  UpperLimit=inf  LowerLimit=150
  Sum : Sum  Inputs=|++
  Power : Outport  VectorParamsAs1DForOutWhenUnconnected=off
  wires:
  Constant1/1 -> Product/2
  Logical Operator/1 -> Product1/1
  GreaterThan/1 -> Logical Operator/1
  Mode/1 -> GreaterThan/1
  Active/1 -> Logical Operator/2
  Constant/1 -> GreaterThan/2
  Product/1 -> Sum/1
  Constant2/1 -> Sum/2
  Sum/1 -> Saturation/1
  RPM/1 -> Abs/1
  Abs/1 -> Product/1
  Saturation/1 -> Product1/2
  Product1/1 -> Power/1

== matlab function Main_Sim/power/input_power/solar_panel_power ==
  data: sc2sun_body_unit input; power_gen_W output; simParams parameter; diodes_A output
function [power_gen_W,diodes_A] = get_power_gen(sc2sun_body_unit,simParams)
%GET_POWER_GEN
% 
% get_power_gen(sc2sun_body_unit,simParams) computes the total power being
% generated by the solar panels located on each of face. Assumes power
% generation is proportional to the square of the cosine of the incidence 
% angle to the sun, and can generate a maximum of 'maxPower' for each face.
%
% Assumes there are solar panels on all 6 sides of cuboid s/c, but fewer
% faces can be modeled by setting the 'maxPower' of those faces to zero.
% ORDER OF FACES: [ +x, -x, +y, -y, +z, -z ]
%
% This function also outputs the current reading from the photodiode on
% each face in Amps as diodes_A
%
% T. Reynolds
%#codegen

power_gen_W = zeros(6,1);
diodes_A    = zeros(6,1);
normals     = simParams.sensors.solar_panels.normals;
maxPower    = simParams.sensors.solar_panels.maxPower;
I_out_ApW   = simParams.sensors.photodiodes.I_out_ApW;

for k = 1:6
   % compute cos(incidence)
   sdotf = dot(normals(:,k),sc2sun_body_unit);
   cinc  = saturate(sdotf);
   incidence = acos(cinc);
   
   if incidence > 0.698132 % greater than 40 degrees
       factor = (-0.369 * cinc^3) + (0.637 * cinc^2) + (0.75 * cinc) -0.015;
   else
       factor = cinc;
   end
       
   if factor < 0
       factor = 0;
   end
   % compute power generated on ith face
   power_gen_W(k) = maxPower(k) * factor; %* cinc * cinc;
   
   % compute photodiode current
   diodes_A(k) = power_gen_W(k) * I_out_ApW; 
end

end

function y = saturate(x)
    if( x < 0 )
        y = 0.0;
    elseif( x >= 1.0 )
        y = 1.0;
    else
        y = x;
    end
end
